simulink model "Simple_non_control"  (R2019a)
settings: Solver=VariableStepAuto  StartTime=0.0  StopTime=10.0  RelTol=1e-3
settings Model: Creator=martin  LastModifiedBy=martin

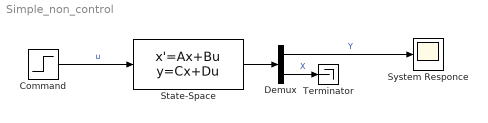
== system Simple_non_control ==
  Command : Step  SampleTime=0
  Demux : Demux  Outputs=2
  State-Space : StateSpace  InitialCondition=0
  System Responce : Scope
  Terminator : Terminator
  wires:
  State-Space/1 -> Demux/1
  Demux/1 -> System Responce/1  "Y"
  Command/1 -> State-Space/1  "u"
  Demux/2 -> Terminator/1  "X"
